simulink subsystem "park_inversa"  (R2020a)
settings: Solver=VariableStepAuto  StartTime=0.0  StopTime=10.0  RelTol=1e-3
settings Model: Creator=Ferran  LastModifiedBy=Ferran

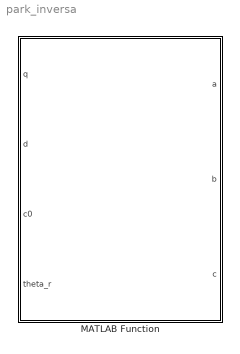
== system park_inversa ==
  MATLAB Function : MATLAB Function  TreatAsAtomicUnit=on

== matlab function park_inversa/MATLAB Function ==
  data: q input; a output; d input; c0 input; theta_r input; b output; c output
function [a,b,c] = TPark_inversa(q,d,c0,theta_r)
    fqd0 = [q;d;c0];
    T = [cos(theta_r)               sin(theta_r)            1;
        cos(theta_r - (2*pi)/3)    sin(theta_r - (2*pi)/3) 1;
        cos(theta_r + (2*pi)/3)    sin(theta_r + (2*pi)/3) 1];
    
    fabc = T*fqd0;
    
    a = fabc(1);
    b = fabc(2);
    c = fabc(3);
end
